simulink model "sl_ex11"  (R2014a)
settings: Solver=ode45  StartTime=0.0  StopTime=10.0  RelTol=1e-3
settings Model: Creator=liang  LastModifiedBy=liang

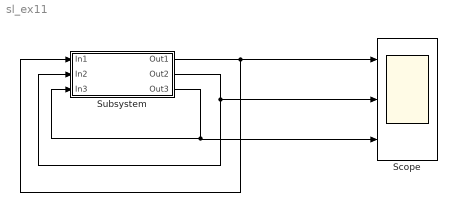
== system sl_ex11 ==
  Scope : Scope  NumInputPorts=3
      settings: YMin=-5~-5~-5  YMax=5~5~5
  Subsystem : Subsystem
  wires:
  Subsystem/1(Out1) -> Scope/1, Subsystem/1(In1)
  Subsystem/3(Out3) -> Scope/3, Subsystem/3(In3)
  Subsystem/2(Out2) -> Scope/2, Subsystem/2(In2)

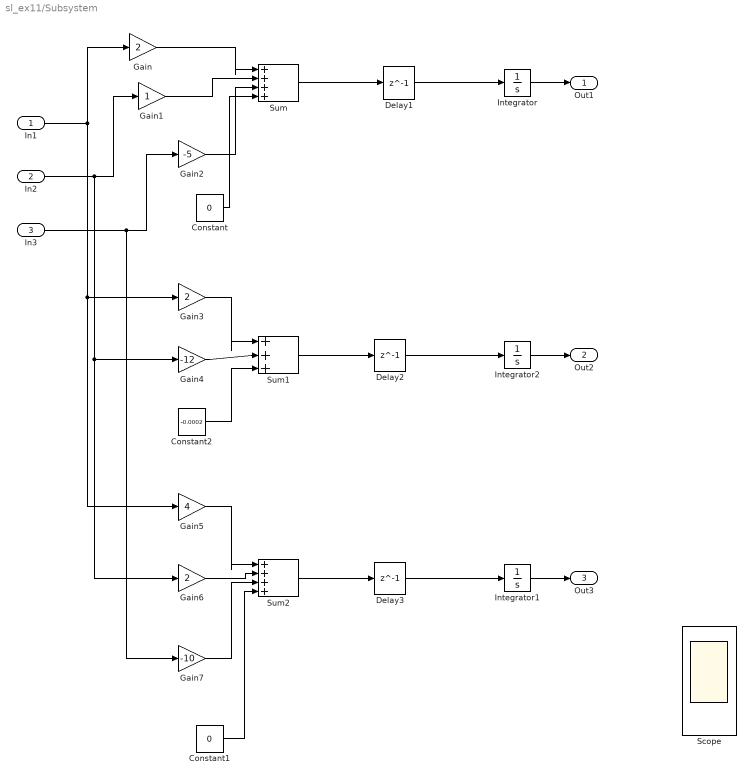
== system sl_ex11/Subsystem ==
  In1 : Inport
  In2 : Inport  Port=2
  In3 : Inport  Port=3
  Constant : Constant  Value=0
  Constant1 : Constant  Value=0
  Constant2 : Constant  Value=-0.0002
  Delay1 : Delay  DelayLength=1  SampleTime=0.01
  Delay2 : Delay  DelayLength=1  SampleTime=0.01
  Delay3 : Delay  DelayLength=1  SampleTime=0.01
  Gain : Gain  Gain=2
  Gain1 : Gain
  Gain2 : Gain  Gain=-5
  Gain3 : Gain  Gain=2
  Gain4 : Gain  Gain=-12
  Gain5 : Gain  Gain=4
  Gain6 : Gain  Gain=2
  Gain7 : Gain  Gain=-10
  Integrator : Integrator  InitialCondition=0.3617
  Integrator1 : Integrator  InitialCondition=0.7234
  Integrator2 : Integrator  InitialCondition=-0.1064
  Scope : Scope
  Sum : Sum  Inputs=|++++
  Sum1 : Sum  Inputs=|+++
  Sum2 : Sum  Inputs=|++++
  Out1 : Outport
  Out2 : Outport  Port=2
  Out3 : Outport  Port=3
  wires:
  Integrator/1 -> Out1/1
  Integrator2/1 -> Out2/1
  Integrator1/1 -> Out3/1
  Sum/1 -> Delay1/1
  In1/1 -> Gain5/1, Gain3/1, Gain/1
  Gain/1 -> Sum/1
  In2/1 -> Gain6/1, Gain4/1, Gain1/1
  Gain1/1 -> Sum/2
  In3/1 -> Gain7/1, Gain2/1
  Gain2/1 -> Sum/3
  Sum1/1 -> Delay2/1
  Gain3/1 -> Sum1/1
  Gain4/1 -> Sum1/2
  Gain5/1 -> Sum2/1
  Gain6/1 -> Sum2/2
  Gain7/1 -> Sum2/3
  Sum2/1 -> Delay3/1
  Delay1/1 -> Integrator/1
  Delay2/1 -> Integrator2/1
  Delay3/1 -> Integrator1/1
  Constant/1 -> Sum/4
  Constant1/1 -> Sum2/4
  Constant2/1 -> Sum1/3
